simulink model "BLDC_Lun"  (R2021b)
settings: Solver=FixedStepAuto  StartTime=0.0  StopTime=10  FixedStep=1e-4  RelTol=1e-4
model workspace (MAT data in the model file):
  f = Simulink.Signal
  f.DataType = 'single'
  f.Dimensions = 1
  f.DimensionsMode = 'auto'
  f.Complexity = 'real'
  f.SampleTime = -1
  f.SamplingMode = 'auto'
  f.InitialValue = '0.1827'
undefined symbols (not defined in the file): curr_d_ki, curr_d_kp, curr_q_ki, curr_q_kp, DiscIntNeverNeededParam, flux, G1, G2, L, Pn, Rs, sigbuilder_block, spd_ki, spd_kp, Tpwm, Ts, Udc
libraries: slpidlib x4, simulink x2, mcbplantlib x1, autolibpmsmexterior x1
settings Model: DataDictionary=BLDC_Lun.sldd  PacingRate=0.630000  Creator=张豪  LastModifiedBy=张豪
settings OptimizationCC: DefaultParameterBehavior=Inlined  UseDivisionForNetSlopeComputation=on  GainParamInheritBuiltInType=on  UseFloatMulNetSlope=on  InlineInvariantSignals=on  PassReuseOutputArgsAs=Individual arguments  ZeroExternalMemoryAtStartup=off  ZeroInternalMemoryAtStartup=off  NoFixptDivByZeroProtection=on  EfficientFloat2IntCast=on  LifeSpan=1  OptimizeBlockOrder=speed  DifferentSizesBufferReuse=on  EfficientTunableParamExpr=on
settings DebuggingCC: ParameterTunabilityLossMsg=error
settings HardwareCC: ProdBitPerPointer=32  ProdBitPerSizeT=32  ProdBitPerPtrDiffT=32  ProdLargestAtomicInteger=Long  ProdLargestAtomicFloat=Double  ProdWordSize=32  ProdLongLongMode=on  ProdHWDeviceType=ARM Compatible->ARM Cortex-M
settings SFSimCC: MATLABDynamicMemAlloc=off
settings RTWCC: Description=Embedded Coder  SystemTargetFile=ert.tlc  GenCodeOnly=on  TemplateMakefile=ert_default_tmf  GenerateReport=on  LaunchReport=on  GenerateCodeReplacementReport=on
settings CodeAppCC: ForceParamTrailComments=on  IgnoreCustomStorageClasses=off  OperatorAnnotations=on  SimulinkDataObjDesc=on  SFDataObjDesc=on  CustomSymbolStrGlobalVar=rt$N$M  CustomSymbolStrType=$N$M  CustomSymbolStrFcn=$N$M$F  CustomSymbolStrMacro=$N$M  InsertBlockDesc=on
settings ERTTargetCC: TargetLangStandard=C99 (ISO)  CodeReplacementLibrary=ARM Cortex-M  GenerateSampleERTMain=on  IncludeMdlTerminateFcn=off  CombineSignalStateStructs=on  SupportComplex=off  SupportNonInlinedSFcns=on  InlinedParameterPlacement=NonHierarchical  ERTCustomFileTemplate=example_file_process.tlc  ERTFilePackagingFormat=CompactWithDataFile

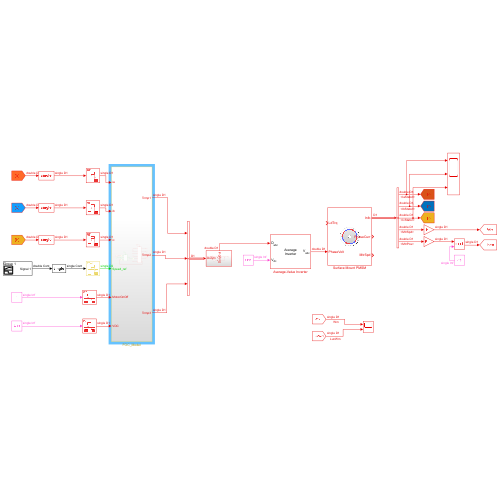
[thumbnail: Simulink's stored preview of the top-level diagram]
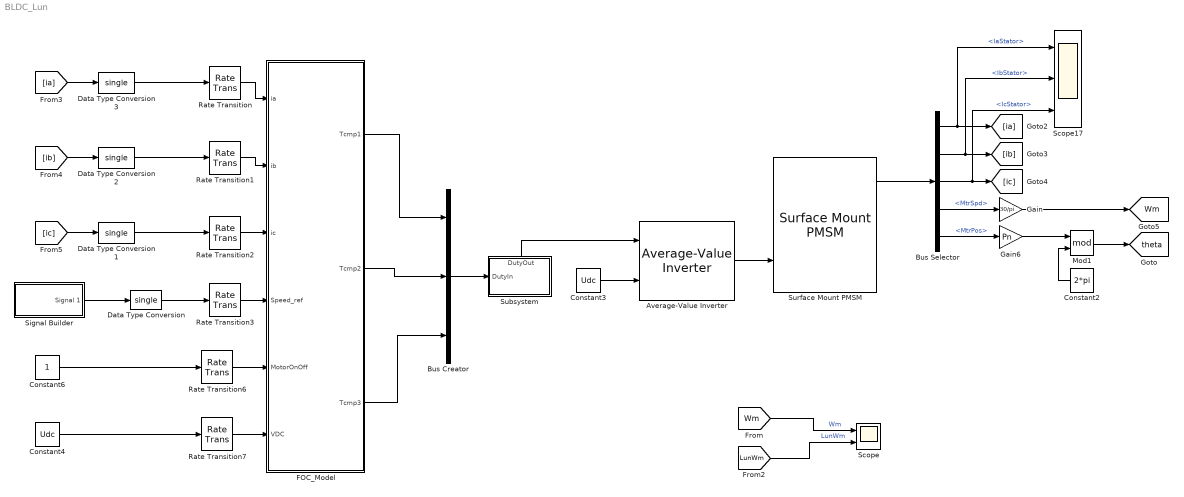
== system BLDC_Lun ==
  Average-Value Inverter : mcbplantlib/Average-Value Inverter
  Bus Creator : BusCreator  Inputs=3
  Bus Selector : BusSelector  OutputSignals=IaStator,IbStator,IcStator,MtrSpd,MtrPos
  Constant2 : Constant  Value=2*pi  OutDataTypeStr=single
  Constant3 : Constant  Value=Udc
  Constant4 : Constant  Value=Udc  OutDataTypeStr=single
  Constant6 : Constant  OutDataTypeStr=single
  Data Type Conversion{,1..3} (4 alike) : DataTypeConversion  OutDataTypeStr=single
  FOC_Model : Subsystem  SystemSampleTime=5e-5
  Gain : Gain  Gain=30/pi  OutDataTypeStr=single
  Gain6 : Gain  Gain=Pn  OutDataTypeStr=single
  Mod1 : Math  Operator=mod  OutputSignalType=real  SaturateOnIntegerOverflow=on
  Rate Transition{,1..3,6..7} (6 alike) : RateTransition
  Scope : Scope  NumInputPorts=2
  Scope17 : Scope  NumInputPorts=3
  Signal Builder : Subsystem  Tag=STV Subsys  LoadFcn=sigbuilder_block('load');  StartFcn=sigbuilder_block('start');  StopFcn=sigbuilder_block('stop');  ClipboardFcn=sigbuilder_block('clipboard');  mask(Sigbuilder block){tuvar=[0:10]}
      mask help: Simulink:masks:SigbuilderBlock_MD
      mask init:
      | if ~strcmp(get_param(bdroot(gcbh),'SimulationStatus'),'stopped') tuvar = sigbuilder_block('maskInit'); end
      settings: CopyFcn=sigbuilder_block('copy');  DeleteFcn=sigbuilder_block('delete');  ModelCloseFcn=sigbuilder_block('modelClose');  PreSaveFcn=sigbuilder_block('preSave');  PauseFcn=sigbuilder_block('pause');  ContinueFcn=sigbuilder_block('continue');  NameChangeFcn=sigbuilder_block('namechange');  OpenFcn=sigbuilder_block('open',[437.6 199.2 550.4 400 ]);  CloseFcn=sigbuilder_block('close');
      mask Display: plot(0, 0, 100, 100,[2, 2, 32, 32, 2], [68, 8, 8, 68, 68],[32, 2], [38, 38], [32, 19, 2],[53, 60, 44], [32, 17, 17, 2],[16, 16, 31, 31]);txt = getActiveGroup(gcbh);text(2, 100, txt,'verticalAlignment', 'top');
  Subsystem : Subsystem
      settings: PortSchema="{\"entries\":[{\"content\":{\"sides\":[{\"content\":{\"connectorIds\":[\"In1\"]},\"type\":\"ConnectorPlacement.EquallySpacedRectSide\",\"uuid\":\"8ccc51de-fa2a-4900-80a3-4cdf9aa76f01\"},{\"content\":{\"connectorIds\":[],\"side\":\"RIGHT\"},\"type\":\"ConnectorPlacement.EquallySpacedRectSide\",\"uuid\":\"32c06e0d-3f1d-4948-af96-e310e54308a0\"},{\"content\":{\"connectorIds\":[\"Out1\"],\"side\":\"TOP\"},\"type\":\"ConnectorPlacement.EquallySpacedRectSide\",\"uuid\":\"a9066067-2c54-42a8-b4d7-fb86ac71b860\"}]},\"type\":\"ConnectorPlacement.EquallySpacedConnector\",\"uuid\":\"e4576975-acad-4e16-822f-2c2e7f23d7a7\"}],\"packageUris\":[\"http://schema.mathworks.com/mf0/Connector/R2020b\"],\"version\":\"1.0\"}"
  Surface Mount PMSM : autolibpmsmexterior/Surface Mount PMSM  port_config=Torque  sim_type=Discrete  Ts=1e-4  P=Pn  Rs=Rs  Ldq_=L  KConstText=Permanent flux linkage constant (lambda_pm):  lambda_pm=flux  Ke=0.0059268  Kt=0.061  mechanical=[75e-6, 8e-5, 0]  idq0=[0 0]  theta_init=4/5  omega_init=0  KConst=flux  lambda_pm_calc=flux  RefBlkName='autolibpmsmexterior/Surface Mount PMSM'  aMode=5  Ldq="[0.0017      0.0017]"
      settings: SourceProductBaseCode=PW,DR,MT,UV,VE
  tag scope: Wm=global, theta=global
  wires:
  Gain/1 -> [Wm]
  [ia] -> Data Type Conversion3/1
  [ib] -> Data Type Conversion2/1
  [ic] -> Data Type Conversion1/1
  Subsystem/1(DutyOut) -> Average-Value Inverter/1
  Average-Value Inverter/1 -> Surface Mount PMSM/2
  Constant3/1 -> Average-Value Inverter/2
  Surface Mount PMSM/1 -> Bus Selector/1
  Bus Selector/1 -> Scope17/1, [ia]  "<IaStator>"
  Bus Selector/2 -> Scope17/2, [ib]  "<IbStator>"
  Bus Selector/3 -> Scope17/3, [ic]  "<IcStator>"
  Bus Selector/4 -> Gain/1  "<MtrSpd>"
  Bus Selector/5 -> Gain6/1  "<MtrPos>"
  Bus Creator/1 -> Subsystem/1(DutyIn)
  FOC_Model/1(Tcmp1) -> Bus Creator/1
  FOC_Model/2(Tcmp2) -> Bus Creator/2
  FOC_Model/3(Tcmp3) -> Bus Creator/3
  Data Type Conversion3/1 -> Rate Transition/1
  Data Type Conversion2/1 -> Rate Transition1/1
  Data Type Conversion1/1 -> Rate Transition2/1
  Signal Builder/1(Signal 1) -> Data Type Conversion/1
  Gain6/1 -> Mod1/1
  Constant2/1 -> Mod1/2
  Rate Transition/1 -> FOC_Model/1(ia)
  Rate Transition1/1 -> FOC_Model/2(ib)
  Rate Transition2/1 -> FOC_Model/3(ic)
  Rate Transition3/1 -> FOC_Model/4(Speed_ref)
  Data Type Conversion/1 -> Rate Transition3/1
  Constant4/1 -> Rate Transition7/1
  Rate Transition6/1 -> FOC_Model/5(MotorOnOff)
  Rate Transition7/1 -> FOC_Model/6(VDC)
  Constant6/1 -> Rate Transition6/1
  Mod1/1 -> [theta]
  [Wm] -> Scope/1  "Wm"
  [LunWm] -> Scope/2  "LunWm"

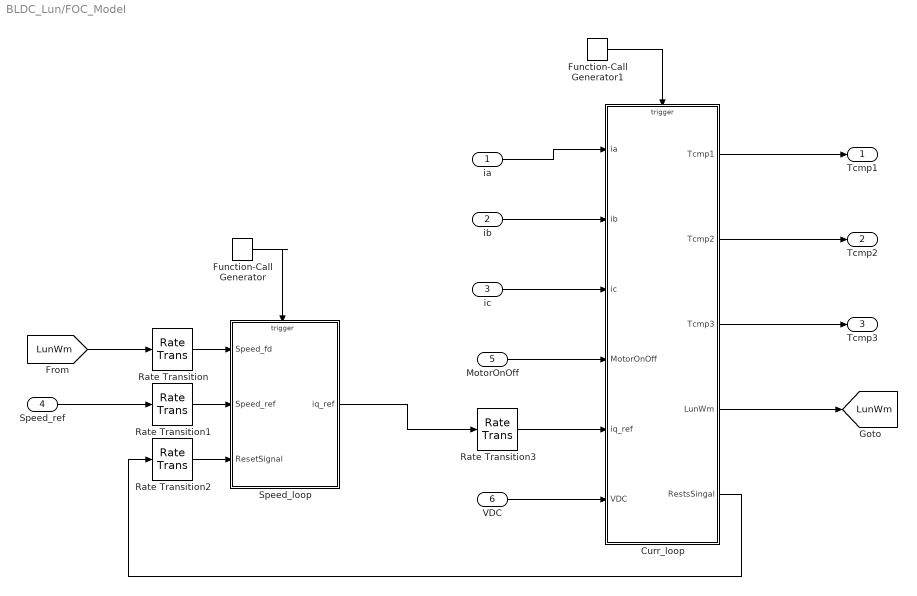
== system BLDC_Lun/FOC_Model ==
  ia : Inport
  ib : Inport  Port=2
  ic : Inport  Port=3
  Speed_ref : Inport  Port=4
  MotorOnOff : Inport  Port=5
  VDC : Inport  Port=6
  Curr_loop : Subsystem  TreatAsAtomicUnit=on
  Function-Call Generator : simulink/Ports & Subsystems/Function-Call Generator  sample_time=1e-3  numberOfIterations=1  DisallowWideOutput=off
  Function-Call Generator1 : simulink/Ports & Subsystems/Function-Call Generator  sample_time=1e-4  numberOfIterations=1  DisallowWideOutput=off
  Rate Transition{,1..3} (4 alike) : RateTransition
  Speed_loop : Subsystem
  Tcmp1 : Outport
  Tcmp2 : Outport  Port=2
  Tcmp3 : Outport  Port=3
  tag scope: LunWm=global
  wires:
  ia/1 -> Curr_loop/1(ia)
  Curr_loop/3(Tcmp3) -> Tcmp3/1
  Curr_loop/1(Tcmp1) -> Tcmp1/1
  ib/1 -> Curr_loop/2(ib)
  Curr_loop/2(Tcmp2) -> Tcmp2/1
  ic/1 -> Curr_loop/3(ic)
  Speed_ref/1 -> Rate Transition1/1
  MotorOnOff/1 -> Curr_loop/4(MotorOnOff)
  VDC/1 -> Curr_loop/6(VDC)
  Curr_loop/4(LunWm) -> [LunWm]
  Rate Transition/1 -> Speed_loop/1(Speed_fd)
  Rate Transition1/1 -> Speed_loop/2(Speed_ref)
  Rate Transition2/1 -> Speed_loop/3(ResetSignal)
  Curr_loop/5(RestsSingal) -> Rate Transition2/1
  [LunWm] -> Rate Transition/1
  Function-Call Generator/1 -> Speed_loop/Trigger
  Rate Transition3/1 -> Curr_loop/5(iq_ref)
  Function-Call Generator1/1 -> Curr_loop/Trigger
  Speed_loop/1(iq_ref) -> Rate Transition3/1

== system BLDC_Lun/Signal Builder ==
  Demux : Demux  Tag=STV Demux  Outputs=1
      settings: DisplayOption=none
  FromWs : FromWorkspace  Tag=STV FromWs  VariableName=tuvar
      SigBuilderData=|
      | common.afterFinalStr = 'Extrapolate'
      | common.sampleTime = 0
      | dataSet.timeRange = [0 10]
      | dataSet.name = 'Group 1'
      | sbobj.Groups.Name = 'Group 1'
      | sbobj.Groups.Signals.Name = 'Signal 1'
      | sbobj.Groups.Signals.XData = [0 4 4 7 7 10]
      | sbobj.Groups.Signals.YData = [680 680 1020 1020 1200 1200]
  Signal 1 : Outport  Tag=STV Outport
  wires:
  Demux/1 -> Signal 1/1
  FromWs/1 -> Demux/1

== system BLDC_Lun/Subsystem ==
  DutyIn : Inport
  Constant : Constant  Value=0.5  SampleTime=-1
  Gain : Gain  Gain=1/8000  ParamDataTypeStr=single
  Gain1 : Gain  Gain=-1
  Sum : Sum  Inputs=|+-
  Sum1 : Sum  Inputs=|++
  DutyOut : Outport
  wires:
  Sum/1 -> Gain1/1
  Constant/1 -> Sum1/2, Sum/2
  DutyIn/1 -> Gain/1
  Gain1/1 -> Sum1/1
  Sum1/1 -> DutyOut/1
  Gain/1 -> Sum/1

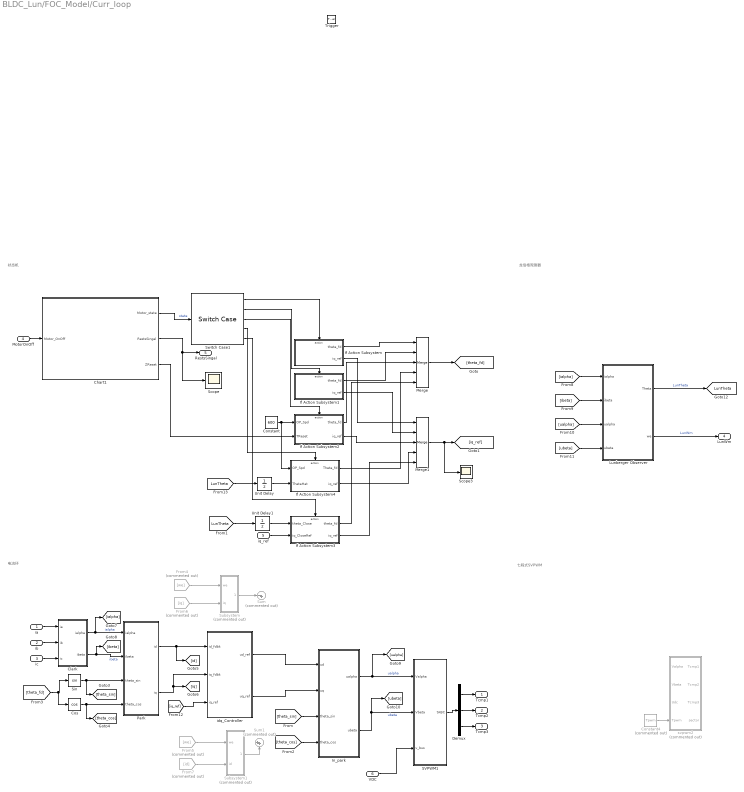
== system BLDC_Lun/FOC_Model/Curr_loop ==
  note: 七段式SVPWM
  note: 电流环
  note: 龙伯格观测器
  note: 状态机
  ia : Inport  OutDataTypeStr=single
  ib : Inport  Port=2  OutDataTypeStr=single
  ic : Inport  Port=3  OutDataTypeStr=single
  MotorOnOff : Inport  Port=4
  iq_ref : Inport  Port=5  OutDataTypeStr=single
  VDC : Inport  Port=6
  Trigger : TriggerPort  TriggerType=function-call  VariantControl=(inherit)  PortDimensions=1
  Chart1 : Stateflow chart  TreatAsAtomicUnit=on
  Clark : Subsystem  TreatAsAtomicUnit=on
  Constant : Constant  Value=600  OutDataTypeStr=int32
  Constant4 : Constant  Commented=on  Value=Tpwm  OutDataTypeStr=single
  Cos : Trigonometry  Operator=cos
  Demux : Demux  Outputs=3
  From4 : From  Commented=on  GotoTag=we
  From5 : From  Commented=on  GotoTag=we
  From6 : From  Commented=on  GotoTag=iq
  From7 : From  Commented=on  GotoTag=id
  If Action Subsystem : Subsystem  TreatAsAtomicUnit=on
  If Action Subsystem1 : Subsystem  TreatAsAtomicUnit=on
  If Action Subsystem2 : Subsystem  TreatAsAtomicUnit=on
  If Action Subsystem3 : Subsystem  TreatAsAtomicUnit=on
  If Action Subsystem4 : Subsystem  TreatAsAtomicUnit=on
  In_park : Subsystem  TreatAsAtomicUnit=on
  Lunberger Observer : Subsystem  TreatAsAtomicUnit=on
  Merge : Merge  Inputs=5
  Merge1 : Merge  Inputs=5
  Park : Subsystem  TreatAsAtomicUnit=on
  SVPWM1 : Subsystem  TreatAsAtomicUnit=on
  Scope : Scope
  Scope3 : Scope
  Sin : Trigonometry
  Subsystem : Subsystem  Commented=on
  Subsystem1 : Subsystem  Commented=on
  Sum : Sum  Commented=on  Inputs=|-+
  Sum1 : Sum  Commented=on  Inputs=|++
  Switch Case1 : SwitchCase  CaseConditions={1,2,3,4,5}  ShowDefaultCase=off
  Unit Delay : UnitDelay  SampleTime=-1  HasFrameUpgradeWarning=on
  Unit Delay1 : UnitDelay  SampleTime=-1  HasFrameUpgradeWarning=on
  idq_Controller : Subsystem
  svpwm2 : MATLAB Function  Commented=on  TreatAsAtomicUnit=on
  Tcmp1 : Outport
  Tcmp2 : Outport  Port=2
  Tcmp3 : Outport  Port=3
  LunWm : Outport  Port=4
  RestsSingal : Outport  Port=5
  tag scope: LunTheta=global
  wires:
  [iq_ref] -> idq_Controller/3(iq_ref)
  Clark/2(ibeta) -> [ibeta], Park/2(ibeta)  "ibeta"
  Park/1(id) -> [id], idq_Controller/1(id_fdbk)
  ib/1 -> Clark/2(ib)
  ia/1 -> Clark/1(ia)
  Clark/1(ialpha) -> [ialpha], Park/1(ialpha)  "ialpha"
  VDC/1 -> SVPWM1/3(v_bus)
  Park/2(iq) -> [iq], idq_Controller/2(iq_fdbk)
  Constant4/1 -> svpwm2/4(Tpwm)
  ic/1 -> Clark/3(ic)
  SVPWM1/1(tABC) -> Demux/1
  Demux/1 -> Tcmp1/1
  Demux/2 -> Tcmp2/1
  Demux/3 -> Tcmp3/1
  In_park/1(ualpha) -> [ualpha], SVPWM1/1(Valpha)  "ualpha"
  In_park/2(ubeta) -> [ubeta], SVPWM1/2(Vbeta)  "ubeta"
  MotorOnOff/1 -> Chart1/1(Motor_OnOff)
  Chart1/1(Motor_state) -> Switch Case1/1  "state"
  Switch Case1/1 -> If Action Subsystem/Action
  Switch Case1/2 -> If Action Subsystem1/Action
  Switch Case1/3 -> If Action Subsystem2/Action
  iq_ref/1 -> If Action Subsystem3/2(iq_CloseRef)
  Constant/1 -> If Action Subsystem4/1(OP_Spd), If Action Subsystem2/1(OP_Spd)
  Chart1/2(RestsSingal) -> Scope/1, RestsSingal/1
  If Action Subsystem/1(theta_fd) -> Merge/1
  If Action Subsystem1/1(theta_fd) -> Merge/2
  If Action Subsystem2/1(theta_fd) -> Merge/3
  If Action Subsystem/2(iq_ref) -> Merge1/1
  If Action Subsystem1/2(iq_ref) -> Merge1/2
  If Action Subsystem2/2(iq_ref) -> Merge1/3
  Merge/1 -> [theta_fd]
  Merge1/1 -> Scope3/1, [iq_ref]
  [LunTheta] -> Unit Delay1/1
  Subsystem/1(Out1) -> Sum/1
  Cos/1 -> [theta_cos], Park/4(theta_cos)
  Sin/1 -> Park/3(theta_sin), [theta_sin]
  Subsystem1/1(Out1) -> Sum1/2
  [theta_sin] -> In_park/3(theta_sin)
  [theta_cos] -> In_park/4(theta_cos)
  From4/1 -> Subsystem/1(we)
  From5/1 -> Subsystem1/1(we)
  From6/1 -> Subsystem/2(iq)
  From7/1 -> Subsystem1/2(id)
  [ialpha] -> Lunberger Observer/1(ialpha)
  [ibeta] -> Lunberger Observer/2(ibeta)
  [ualpha] -> Lunberger Observer/3(ualpha)
  [ubeta] -> Lunberger Observer/4(ubeta)
  Chart1/3(ZReset) -> If Action Subsystem2/2(TReset)
  [theta_fd] -> Cos/1, Sin/1
  idq_Controller/2(uq_ref) -> In_park/2(uq)
  idq_Controller/1(ud_ref) -> In_park/1(ud)
  Switch Case1/4 -> If Action Subsystem4/Action
  Switch Case1/5 -> If Action Subsystem3/Action
  If Action Subsystem3/1(theta_fd) -> Merge/5
  If Action Subsystem3/2(iq_ref) -> Merge1/5
  If Action Subsystem4/1(Theta_fd) -> Merge/4
  If Action Subsystem4/2(iq_ref) -> Merge1/4
  Lunberger Observer/1(Theta) -> [LunTheta]  "LunTheta"
  Lunberger Observer/2(we) -> LunWm/1  "LunWm"
  [LunTheta] -> Unit Delay/1
  Unit Delay/1 -> If Action Subsystem4/2(ThetaHat)
  Unit Delay1/1 -> If Action Subsystem3/1(theta_Close)

== system BLDC_Lun/FOC_Model/Speed_loop ==
  Speed_fd : Inport  OutDataTypeStr=single  PortDimensions=1
  Speed_ref : Inport  Port=2  OutDataTypeStr=single  PortDimensions=1
  ResetSignal : Inport  Port=3
  Trigger : TriggerPort  TriggerType=function-call  VariantControl=(inherit)  PortDimensions=1
  PID Controller3 : slpidlib/PID Controller  Controller=PI  Form=Parallel  TimeDomain=Discrete-time  UseExternalTs=off  SampleTime=-1  IntegratorMethod=Forward Euler  FilterMethod=Forward Euler  ControllerParametersSource=internal  P=spd_kp  I=spd_ki  D=0  UseFilter=on  N=100  TunerSelectOption=Transfer Function Based (PID Tuner App)  InitialConditionSource=internal  InitialConditionForIntegrator=0  InitialConditionForFilter=0  DifferentiatorICPrevScaledInput=0  ExternalReset=rising  TrackingMode=off  Kt=1  LimitOutput=on  SatLimitsSource=internal  UpperSaturationLimit=3  LowerSaturationLimit=-3  LinearizeAsGain=on  AntiWindupMode=clamping  Kb=0.013  PGainOutDataTypeStr=single  PProdOutDataTypeStr=single  POutMin=[]  POutMax=[]  IGainOutDataTypeStr=single  IProdOutDataTypeStr=single  IOutMin=[]  IOutMax=[]  DOutMin=[]  DOutMax=[]  NOutMin=[]  NOutMax=[]  SumOutDataTypeStr=single  SumOutMin=[]  SumOutMax=[]  SaturationOutDataTypeStr=single  SaturationOutMin=[]  SaturationOutMax=[]  PParamMin=[]  PParamMax=[]  IParamMin=[]  IParamMax=[]  DParamMin=[]  DParamMax=[]  NParamMin=[]  NParamMax=[]  KbParamMin=[]  KbParamMax=[]  KtParamMin=[]  KtParamMax=[]  KbOutMin=[]  KbOutMax=[]  KtOutMin=[]  KtOutMax=[]  IntegratorOutMin=[]  IntegratorOutMax=[]  FilterOutMin=[]  FilterOutMax=[]  SumI1OutMin=[]  SumI1OutMax=[]  SumI2OutMin=[]  SumI2OutMax=[]  SumI3OutMin=[]  SumI3OutMax=[]  SumI4OutMin=[]  SumI4OutMax=[]  SumDOutMin=[]  SumDOutMax=[]  DifferentiatorOutMin=[]  DifferentiatorOutMax=[]  FilterDiffOutCoefMin=[]  FilterDiffOutCoefMax=[]  ReciprocalOutMin=[]  ReciprocalOutMax=[]  SumDenOutMin=[]  SumDenOutMax=[]  SumNumOutMin=[]  SumNumOutMax=[]  DivideOutMin=[]  DivideOutMax=[]  UdiffTsProdOutMin=[]  UdiffTsProdOutMax=[]  NTsProdOutMin=[]  NTsProdOutMax=[]  UintegralTsProdOutMin=[]  UintegralTsProdOutMax=[]  UngainTsProdOutMin=[]  UngainTsProdOutMax=[]  IntegratorContinuousStateAttributes=''  IntegratorStateMustResolveToSignalObject=off  IntegratorRTWStateStorageClass=Auto  FilterContinuousStateAttributes=''  FilterStateMustResolveToSignalObject=off  FilterRTWStateStorageClass=Auto  ParallelPVariant=InternalParameters  IdealPVariant=Disabled  IVariant=InternalParameters  DVariant=Disabled  IntegratorVariant=Discrete  SatVariant=Enabled  AWVariant=DiscClampingParallel  PCopyVariant=Disabled  TRVariant=Disabled  FdbkBlocksVariant=Forward  IdealPFdbkVariant=Disabled  SatFdbkVariant=Disabled  DerivativeFilterVariant=Disabled  NVariant=Disabled  NCopyVariant=Disabled_SignalSpec  FilterICVariant=Disabled  IntegratorICVariant=InternalICs  ExternalResetVariant=ExternalReset  TRSumVariant=Passthrough  SumFdbkVariant=Disabled  SumVariant=Sum_PI  TsampFilterVariant=InternalTs  TsampNgainVariant=Passthrough  TsampIntegralVariant=Passthrough  ExternalSaturationOutDataTypeStr=single
  Sum2 : Sum  Inputs=|+-  AccumDataTypeStr=single  OutDataTypeStr=single
  iq_ref : Outport
  wires:
  Sum2/1 -> PID Controller3/1
  Speed_ref/1 -> Sum2/1
  Speed_fd/1 -> Sum2/2
  PID Controller3/1 -> iq_ref/1
  ResetSignal/1 -> PID Controller3/2

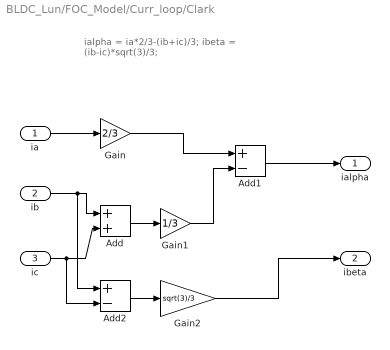
== system BLDC_Lun/FOC_Model/Curr_loop/Clark ==
  note: ialpha = ia*2/3-(ib+ic)/3;
      | ibeta = (ib-ic)*sqrt(3)/3;
  ia : Inport  OutDataTypeStr=single
  ib : Inport  Port=2  OutDataTypeStr=single
  ic : Inport  Port=3  OutDataTypeStr=single
  Add : Sum  AccumDataTypeStr=single  OutDataTypeStr=single
  Add1 : Sum  Inputs=+-  AccumDataTypeStr=single  OutDataTypeStr=single
  Add2 : Sum  Inputs=+-  AccumDataTypeStr=single  OutDataTypeStr=single
  Gain : Gain  Gain=2/3  ParamDataTypeStr=single
  Gain1 : Gain  Gain=1/3  ParamDataTypeStr=single
  Gain2 : Gain  Gain=sqrt(3)/3  ParamDataTypeStr=single
  ialpha : Outport  OutDataTypeStr=single
  ibeta : Outport  Port=2  OutDataTypeStr=single
  wires:
  ia/1 -> Gain/1
  ib/1 -> Add2/1, Add/1
  ic/1 -> Add2/2, Add/2
  Add/1 -> Gain1/1
  Gain/1 -> Add1/1
  Gain1/1 -> Add1/2
  Add1/1 -> ialpha/1
  Add2/1 -> Gain2/1
  Gain2/1 -> ibeta/1

== system BLDC_Lun/FOC_Model/Curr_loop/If Action Subsystem ==
  Action Port : ActionPort  ActionPortLabel=case [ 1 ]:
  Constant : Constant  Value=0  OutDataTypeStr=single
  Constant1 : Constant  Value=0  OutDataTypeStr=single
  theta_fd : Outport
  iq_ref : Outport  Port=2
  wires:
  Constant/1 -> theta_fd/1
  Constant1/1 -> iq_ref/1

== system BLDC_Lun/FOC_Model/Curr_loop/If Action Subsystem1 ==
  Action Port : ActionPort  ActionPortLabel=case [ 2 ]:
  Constant : Constant  Value=0  OutDataTypeStr=single
  Constant1 : Constant  OutDataTypeStr=single
  theta_fd : Outport
  iq_ref : Outport  Port=2
  wires:
  Constant1/1 -> iq_ref/1
  Constant/1 -> theta_fd/1

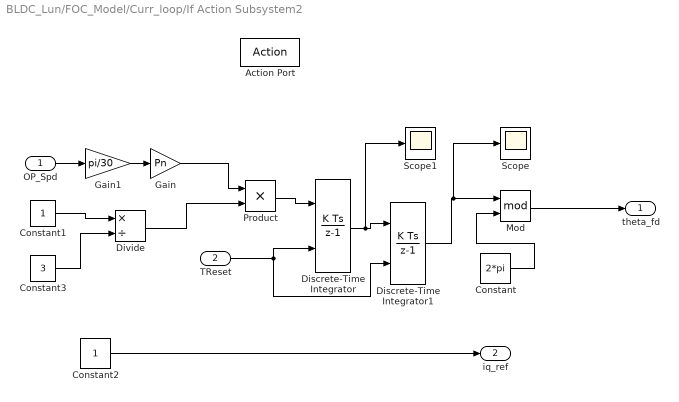
== system BLDC_Lun/FOC_Model/Curr_loop/If Action Subsystem2 ==
  OP_Spd : Inport  OutDataTypeStr=int32  PortDimensions=1
  TReset : Inport  Port=2
  Action Port : ActionPort  ActionPortLabel=case [ 3 ]:
  Constant : Constant  Value=2*pi  OutDataTypeStr=single
  Constant1 : Constant  OutDataTypeStr=single
  Constant2 : Constant  OutDataTypeStr=single
  Constant3 : Constant  Value=3  OutDataTypeStr=single
  Discrete-Time Integrator : DiscreteIntegrator  ExternalReset=rising  SampleTime=-1  ICPrevOutput=DiscIntNeverNeededParam  ICPrevScaledInput=DiscIntNeverNeededParam
  Discrete-Time Integrator1 : DiscreteIntegrator  ExternalReset=rising  SampleTime=-1  ICPrevOutput=DiscIntNeverNeededParam  ICPrevScaledInput=DiscIntNeverNeededParam
  Divide : Product  Inputs=*/  OutDataTypeStr=single
  Gain : Gain  Gain=Pn
  Gain1 : Gain  Gain=pi/30  OutDataTypeStr=single
  Mod : Math  Operator=mod  SaturateOnIntegerOverflow=on
  Product : Product  OutDataTypeStr=single
  Scope : Scope
  Scope1 : Scope
  theta_fd : Outport
  iq_ref : Outport  Port=2
  wires:
  Gain1/1 -> Gain/1
  Constant1/1 -> Divide/1
  Gain/1 -> Product/1
  Constant/1 -> Mod/2
  Discrete-Time Integrator1/1 -> Scope/1, Mod/1
  Mod/1 -> theta_fd/1
  Constant3/1 -> Divide/2
  Constant2/1 -> iq_ref/1
  Divide/1 -> Product/2
  Product/1 -> Discrete-Time Integrator/1
  OP_Spd/1 -> Gain1/1
  TReset/1 -> Discrete-Time Integrator/2, Discrete-Time Integrator1/2
  Discrete-Time Integrator/1 -> Scope1/1, Discrete-Time Integrator1/1

== system BLDC_Lun/FOC_Model/Curr_loop/If Action Subsystem3 ==
  theta_Close : Inport
  iq_CloseRef : Inport  Port=2
  Action Port : ActionPort  ActionPortLabel=case [ 5 ]:
  theta_fd : Outport
  iq_ref : Outport  Port=2
  wires:
  iq_CloseRef/1 -> iq_ref/1
  theta_Close/1 -> theta_fd/1

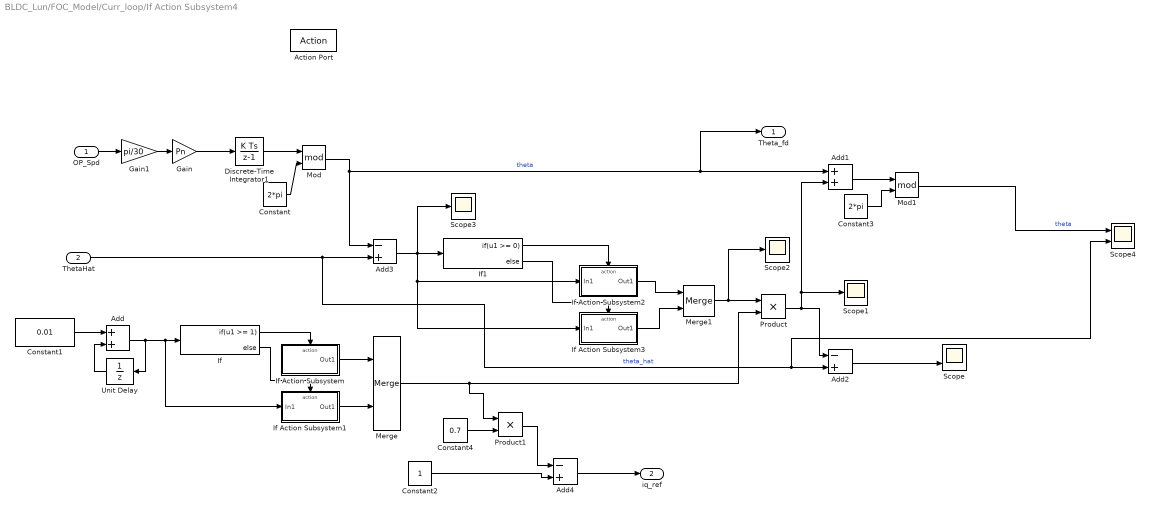
== system BLDC_Lun/FOC_Model/Curr_loop/If Action Subsystem4 ==
  OP_Spd : Inport  OutDataTypeStr=int32  PortDimensions=1
  ThetaHat : Inport  Port=2
  Action Port : ActionPort  ActionPortLabel=case [ 4 ]:
  Add : Sum
  Add1 : Sum
  Add2 : Sum  Inputs=-+
  Add3 : Sum  Inputs=-+
  Add4 : Sum  Inputs=-+
  Constant : Constant  Value=2*pi  OutDataTypeStr=single
  Constant1 : Constant  Value=0.01  OutDataTypeStr=single
  Constant2 : Constant  OutDataTypeStr=single
  Constant3 : Constant  Value=2*pi  OutDataTypeStr=single
  Constant4 : Constant  Value=0.7  OutDataTypeStr=single
  Discrete-Time Integrator1 : DiscreteIntegrator  SampleTime=-1  ICPrevOutput=DiscIntNeverNeededParam  ICPrevScaledInput=DiscIntNeverNeededParam
  Gain : Gain  Gain=Pn
  Gain1 : Gain  Gain=pi/30  OutDataTypeStr=single
  If : If  IfExpression=u1 >= 1
  If Action Subsystem : Subsystem  TreatAsAtomicUnit=on
  If Action Subsystem1 : Subsystem  TreatAsAtomicUnit=on
  If Action Subsystem2 : Subsystem  TreatAsAtomicUnit=on
  If Action Subsystem3 : Subsystem  TreatAsAtomicUnit=on
  If1 : If  IfExpression=u1 >= 0
  Merge : Merge
  Merge1 : Merge
  Mod : Math  Operator=mod  SaturateOnIntegerOverflow=on
  Mod1 : Math  Operator=mod  SaturateOnIntegerOverflow=on
  Product : Product
  Product1 : Product
  Scope : Scope  NumInputPorts=2
  Scope1 : Scope
  Scope2 : Scope
  Scope3 : Scope
  Scope4 : Scope  NumInputPorts=2
  Unit Delay : UnitDelay  SampleTime=-1  HasFrameUpgradeWarning=on
  Theta_fd : Outport
  iq_ref : Outport  Port=2
  wires:
  Gain/1 -> Discrete-Time Integrator1/1
  Constant/1 -> Mod/2
  Discrete-Time Integrator1/1 -> Mod/1
  Constant1/1 -> Add/1
  OP_Spd/1 -> Gain1/1
  If/1 -> If Action Subsystem/Action
  Gain1/1 -> Gain/1
  If Action Subsystem1/1(Out1) -> Merge/2
  Unit Delay/1 -> Add/2
  Add/1 -> Unit Delay/1, If/1, If Action Subsystem1/1(In1)
  If Action Subsystem/1(Out1) -> Merge/1
  If/2 -> If Action Subsystem1/Action
  ThetaHat/1 -> Scope4/2, Add2/2, Add3/2  "theta_hat"
  Mod/1 -> Theta_fd/1, Add1/1, Add3/1  "theta"
  Add3/1 -> Scope3/1, If Action Subsystem3/1(In1), If Action Subsystem2/1(In1), If1/1
  If1/1 -> If Action Subsystem2/Action
  If1/2 -> If Action Subsystem3/Action
  If Action Subsystem2/1(Out1) -> Merge1/1
  If Action Subsystem3/1(Out1) -> Merge1/2
  Merge1/1 -> Scope2/1, Product/1
  Merge/1 -> Product1/1, Product/2
  Product/1 -> Add1/2, Scope1/1, Add2/1
  Add2/1 -> Scope/2
  Constant3/1 -> Mod1/2
  Add1/1 -> Mod1/1
  Mod1/1 -> Scope4/1  "theta"
  Constant4/1 -> Product1/2
  Constant2/1 -> Add4/2
  Product1/1 -> Add4/1
  Add4/1 -> iq_ref/1

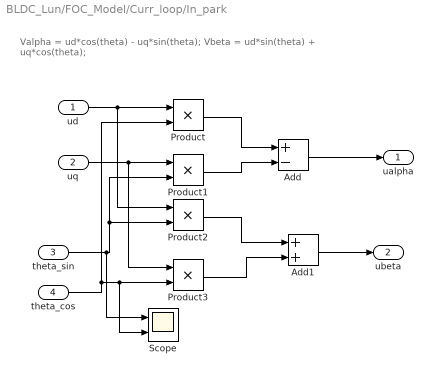
== system BLDC_Lun/FOC_Model/Curr_loop/In_park ==
  note: Valpha = ud*cos(theta) - uq*sin(theta);
      | Vbeta = ud*sin(theta) + uq*cos(theta);
  ud : Inport
  uq : Inport  Port=2
  theta_sin : Inport  Port=3
  theta_cos : Inport  Port=4
  Add : Sum  Inputs=+-
  Add1 : Sum
  Product{,1..3} (4 alike) : Product
  Scope : Scope  NumInputPorts=2
  ualpha : Outport
  ubeta : Outport  Port=2
  wires:
  Add/1 -> ualpha/1
  ud/1 -> Product2/1, Product/1
  theta_cos/1 -> Product/2, Scope/2, Product3/2
  Product/1 -> Add/1
  uq/1 -> Product3/1, Product1/1
  theta_sin/1 -> Scope/1, Product2/2, Product1/2
  Product1/1 -> Add/2
  Product2/1 -> Add1/1
  Product3/1 -> Add1/2
  Add1/1 -> ubeta/1

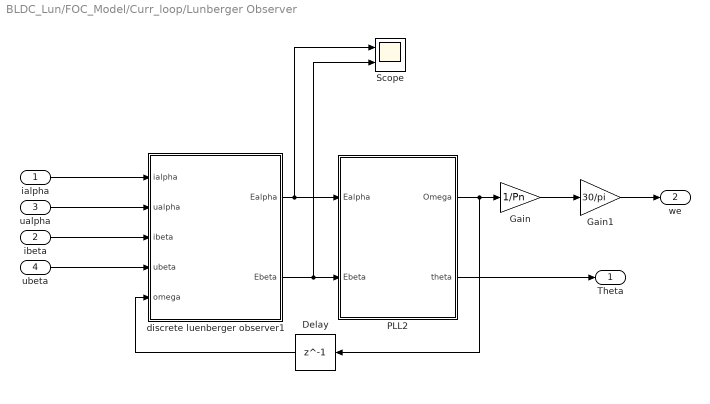
== system BLDC_Lun/FOC_Model/Curr_loop/Lunberger Observer ==
  ialpha : Inport  OutDataTypeStr=single
  ibeta : Inport  Port=2  OutDataTypeStr=single
  ualpha : Inport  Port=3  OutDataTypeStr=single
  ubeta : Inport  Port=4  OutDataTypeStr=single
  Delay : Delay  DelayLength=1  InputProcessing=Columns as channels (frame based)
  Gain : Gain  Gain=1/Pn
  Gain1 : Gain  Gain=30/pi
  PLL2 : Subsystem
  Scope : Scope  NumInputPorts=2
  discrete luenberger observer1 : Subsystem
  Theta : Outport
  we : Outport  Port=2
  wires:
  PLL2/2(theta) -> Theta/1
  ubeta/1 -> discrete luenberger observer1/4(ubeta)
  ibeta/1 -> discrete luenberger observer1/3(ibeta)
  ualpha/1 -> discrete luenberger observer1/2(ualpha)
  ialpha/1 -> discrete luenberger observer1/1(ialpha)
  Delay/1 -> discrete luenberger observer1/5(omega)
  discrete luenberger observer1/1(Ealpha) -> Scope/1, PLL2/1(Ealpha)
  discrete luenberger observer1/2(Ebeta) -> Scope/2, PLL2/2(Ebeta)
  PLL2/1(Omega) -> Gain/1, Delay/1
  Gain/1 -> Gain1/1
  Gain1/1 -> we/1

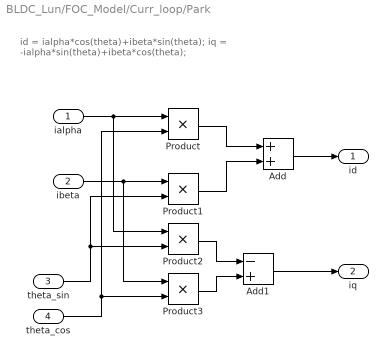
== system BLDC_Lun/FOC_Model/Curr_loop/Park ==
  note: id = ialpha*cos(theta)+ibeta*sin(theta);
      | iq = -ialpha*sin(theta)+ibeta*cos(theta);
  ialpha : Inport  OutDataTypeStr=single
  ibeta : Inport  Port=2  OutDataTypeStr=single
  theta_sin : Inport  Port=3  OutDataTypeStr=single
  theta_cos : Inport  Port=4  OutDataTypeStr=single
  Add : Sum  AccumDataTypeStr=single  OutDataTypeStr=single
  Add1 : Sum  Inputs=-+  AccumDataTypeStr=single  OutDataTypeStr=single
  Product{,1..3} (4 alike) : Product  OutDataTypeStr=single
  id : Outport  OutDataTypeStr=single
  iq : Outport  Port=2  OutDataTypeStr=single
  wires:
  ialpha/1 -> Product2/1, Product/1
  theta_cos/1 -> Product3/2, Product/2
  ibeta/1 -> Product3/1, Product1/1
  theta_sin/1 -> Product2/2, Product1/2
  Product/1 -> Add/1
  Product1/1 -> Add/2
  Add/1 -> id/1
  Product2/1 -> Add1/1
  Product3/1 -> Add1/2
  Add1/1 -> iq/1

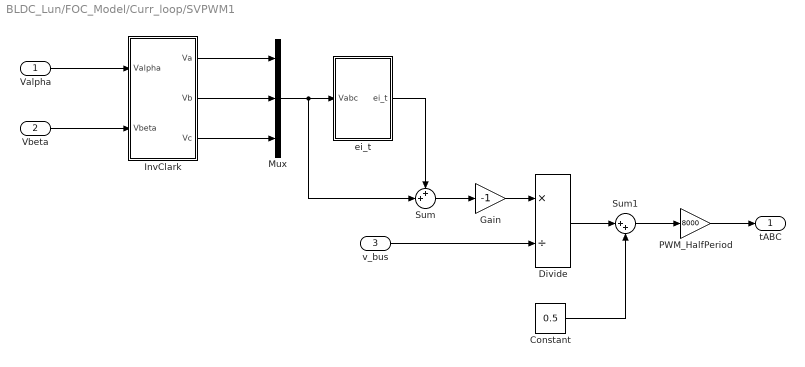
== system BLDC_Lun/FOC_Model/Curr_loop/SVPWM1 ==
  Valpha : Inport  OutDataTypeStr=single
  Vbeta : Inport  Port=2  OutDataTypeStr=single
  v_bus : Inport  Port=3  OutDataTypeStr=single
  Constant : Constant  Value=0.5  OutDataTypeStr=single
  Divide : Product  Inputs=*/  OutDataTypeStr=single
  Gain : Gain  Gain=-1  OutDataTypeStr=single
  InvClark : Subsystem
  Mux : Mux  Inputs=3
  PWM_HalfPeriod : Gain  Gain=8000  OutDataTypeStr=single
  Sum : Sum  Inputs=++|  OutDataTypeStr=single
  Sum1 : Sum  Inputs=|++  OutDataTypeStr=single
  ei_t : Subsystem
  tABC : Outport  OutDataTypeStr=single
  wires:
  Valpha/1 -> InvClark/1(Valpha)
  Vbeta/1 -> InvClark/2(Vbeta)
  ei_t/1(ei_t) -> Sum/1
  InvClark/1(Va) -> Mux/1
  InvClark/2(Vb) -> Mux/2
  InvClark/3(Vc) -> Mux/3
  Sum/1 -> Gain/1
  Mux/1 -> Sum/2, ei_t/1(Vabc)
  Divide/1 -> Sum1/1
  Constant/1 -> Sum1/2
  Sum1/1 -> PWM_HalfPeriod/1
  PWM_HalfPeriod/1 -> tABC/1
  v_bus/1 -> Divide/2
  Gain/1 -> Divide/1

== system BLDC_Lun/FOC_Model/Curr_loop/Subsystem ==
  we : Inport
  iq : Inport  Port=2
  Constant : Constant  Value=L  OutDataTypeStr=single
  Product : Product  Inputs=3
  Out1 : Outport
  wires:
  iq/1 -> Product/2
  we/1 -> Product/1
  Constant/1 -> Product/3
  Product/1 -> Out1/1

== system BLDC_Lun/FOC_Model/Curr_loop/Subsystem1 ==
  we : Inport
  id : Inport  Port=2
  Add : Sum
  Constant : Constant  Value=L  OutDataTypeStr=single
  Constant1 : Constant  Value=flux  OutDataTypeStr=single
  Product : Product
  Product1 : Product
  Out1 : Outport
  wires:
  id/1 -> Product/1
  Constant/1 -> Product/2
  Product/1 -> Add/2
  Constant1/1 -> Add/1
  Product1/1 -> Out1/1
  Add/1 -> Product1/2
  we/1 -> Product1/1

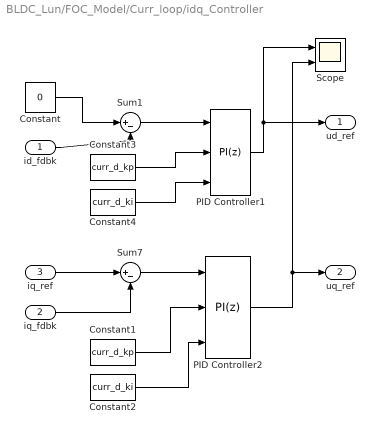
== system BLDC_Lun/FOC_Model/Curr_loop/idq_Controller ==
  id_fdbk : Inport  OutDataTypeStr=single
  iq_fdbk : Inport  Port=2  OutDataTypeStr=single
  iq_ref : Inport  Port=3  OutDataTypeStr=single
  Constant : Constant  Value=0  OutDataTypeStr=single
  Constant1 : Constant  Value=curr_d_kp  OutDataTypeStr=single
  Constant2 : Constant  Value=curr_d_ki  OutDataTypeStr=single
  Constant3 : Constant  Value=curr_d_kp  OutDataTypeStr=single
  Constant4 : Constant  Value=curr_d_ki  OutDataTypeStr=single
  PID Controller1 : slpidlib/PID Controller  Controller=PI  Form=Parallel  TimeDomain=Discrete-time  UseExternalTs=off  SampleTime=-1  IntegratorMethod=Forward Euler  FilterMethod=Forward Euler  ControllerParametersSource=external  P=curr_d_kp  I=curr_d_ki  D=0  UseFilter=on  N=100  TunerSelectOption=Transfer Function Based (PID Tuner App)  InitialConditionSource=internal  InitialConditionForIntegrator=0  InitialConditionForFilter=0  DifferentiatorICPrevScaledInput=0  ExternalReset=none  TrackingMode=off  Kt=1  LimitOutput=on  SatLimitsSource=internal  UpperSaturationLimit=24*0.9/sqrt(3)  LowerSaturationLimit=-24*0.9/sqrt(3)  LinearizeAsGain=on  AntiWindupMode=clamping  Kb=1  PGainOutDataTypeStr=single  PProdOutDataTypeStr=single  POutMin=[]  POutMax=[]  IGainOutDataTypeStr=int16  IProdOutDataTypeStr=int16  IOutMin=[]  IOutMax=[]  DOutMin=[]  DOutMax=[]  NOutMin=[]  NOutMax=[]  SumOutDataTypeStr=single  SumOutMin=[]  SumOutMax=[]  SaturationOutDataTypeStr=single  SaturationOutMin=[]  SaturationOutMax=[]  PParamMin=[]  PParamMax=[]  IParamMin=[]  IParamMax=[]  DParamMin=[]  DParamMax=[]  NParamMin=[]  NParamMax=[]  KbParamMin=[]  KbParamMax=[]  KtParamMin=[]  KtParamMax=[]  KbOutMin=[]  KbOutMax=[]  KtOutMin=[]  KtOutMax=[]  IntegratorOutMin=[]  IntegratorOutMax=[]  FilterOutMin=[]  FilterOutMax=[]  SumI1OutMin=[]  SumI1OutMax=[]  SumI2OutMin=[]  SumI2OutMax=[]  SumI3OutMin=[]  SumI3OutMax=[]  SumI4OutMin=[]  SumI4OutMax=[]  SumDOutMin=[]  SumDOutMax=[]  DifferentiatorOutMin=[]  DifferentiatorOutMax=[]  FilterDiffOutCoefMin=[]  FilterDiffOutCoefMax=[]  ReciprocalOutMin=[]  ReciprocalOutMax=[]  SumDenOutMin=[]  SumDenOutMax=[]  SumNumOutMin=[]  SumNumOutMax=[]  DivideOutMin=[]  DivideOutMax=[]  UdiffTsProdOutMin=[]  UdiffTsProdOutMax=[]  NTsProdOutMin=[]  NTsProdOutMax=[]  UintegralTsProdOutMin=[]  UintegralTsProdOutMax=[]  UngainTsProdOutMin=[]  UngainTsProdOutMax=[]  IntegratorContinuousStateAttributes=''  IntegratorStateMustResolveToSignalObject=off  IntegratorRTWStateStorageClass=Auto  FilterContinuousStateAttributes=''  FilterStateMustResolveToSignalObject=off  FilterRTWStateStorageClass=Auto  ParallelPVariant=ExternalParameters  IdealPVariant=Disabled  IVariant=ExternalParameters  DVariant=Disabled  IntegratorVariant=Discrete  SatVariant=Enabled  AWVariant=DiscClampingParallel  PCopyVariant=Disabled  TRVariant=Disabled  FdbkBlocksVariant=Forward  IdealPFdbkVariant=Disabled  SatFdbkVariant=Disabled  DerivativeFilterVariant=Disabled  NVariant=Disabled  NCopyVariant=Disabled_SignalSpec  FilterICVariant=Disabled  IntegratorICVariant=InternalICs  ExternalResetVariant=Disabled  TRSumVariant=Passthrough  SumFdbkVariant=Disabled  SumVariant=Sum_PI  TsampFilterVariant=InternalTs  TsampNgainVariant=Passthrough  TsampIntegralVariant=Passthrough  ExternalSaturationOutDataTypeStr=Inherit: Same as second input
  PID Controller2 : slpidlib/PID Controller  Controller=PI  Form=Parallel  TimeDomain=Discrete-time  UseExternalTs=off  SampleTime=-1  IntegratorMethod=Forward Euler  FilterMethod=Forward Euler  ControllerParametersSource=external  P=curr_q_kp  I=curr_q_ki  D=0  UseFilter=on  N=100  TunerSelectOption=Transfer Function Based (PID Tuner App)  InitialConditionSource=internal  InitialConditionForIntegrator=0  InitialConditionForFilter=0  DifferentiatorICPrevScaledInput=0  ExternalReset=none  TrackingMode=off  Kt=1  LimitOutput=on  SatLimitsSource=internal  UpperSaturationLimit=24*0.9/sqrt(3)  LowerSaturationLimit=-24*0.9/sqrt(3)  LinearizeAsGain=on  AntiWindupMode=clamping  Kb=1  PGainOutDataTypeStr=single  PProdOutDataTypeStr=single  POutMin=[]  POutMax=[]  IGainOutDataTypeStr=single  IProdOutDataTypeStr=single  IOutMin=[]  IOutMax=[]  DOutMin=[]  DOutMax=[]  NOutMin=[]  NOutMax=[]  SumOutDataTypeStr=single  SumOutMin=[]  SumOutMax=[]  SaturationOutDataTypeStr=single  SaturationOutMin=[]  SaturationOutMax=[]  PParamMin=[]  PParamMax=[]  IParamMin=[]  IParamMax=[]  DParamMin=[]  DParamMax=[]  NParamMin=[]  NParamMax=[]  KbParamMin=[]  KbParamMax=[]  KtParamMin=[]  KtParamMax=[]  KbOutMin=[]  KbOutMax=[]  KtOutMin=[]  KtOutMax=[]  IntegratorOutMin=[]  IntegratorOutMax=[]  FilterOutMin=[]  FilterOutMax=[]  SumI1OutMin=[]  SumI1OutMax=[]  SumI2OutMin=[]  SumI2OutMax=[]  SumI3OutMin=[]  SumI3OutMax=[]  SumI4OutMin=[]  SumI4OutMax=[]  SumDOutMin=[]  SumDOutMax=[]  DifferentiatorOutMin=[]  DifferentiatorOutMax=[]  FilterDiffOutCoefMin=[]  FilterDiffOutCoefMax=[]  ReciprocalOutMin=[]  ReciprocalOutMax=[]  SumDenOutMin=[]  SumDenOutMax=[]  SumNumOutMin=[]  SumNumOutMax=[]  DivideOutMin=[]  DivideOutMax=[]  UdiffTsProdOutMin=[]  UdiffTsProdOutMax=[]  NTsProdOutMin=[]  NTsProdOutMax=[]  UintegralTsProdOutMin=[]  UintegralTsProdOutMax=[]  UngainTsProdOutMin=[]  UngainTsProdOutMax=[]  IntegratorContinuousStateAttributes=''  IntegratorStateMustResolveToSignalObject=off  IntegratorRTWStateStorageClass=Auto  FilterContinuousStateAttributes=''  FilterStateMustResolveToSignalObject=off  FilterRTWStateStorageClass=Auto  ParallelPVariant=ExternalParameters  IdealPVariant=Disabled  IVariant=ExternalParameters  DVariant=Disabled  IntegratorVariant=Discrete  SatVariant=Enabled  AWVariant=DiscClampingParallel  PCopyVariant=Disabled  TRVariant=Disabled  FdbkBlocksVariant=Forward  IdealPFdbkVariant=Disabled  SatFdbkVariant=Disabled  DerivativeFilterVariant=Disabled  NVariant=Disabled  NCopyVariant=Disabled_SignalSpec  FilterICVariant=Disabled  IntegratorICVariant=InternalICs  ExternalResetVariant=Disabled  TRSumVariant=Passthrough  SumFdbkVariant=Disabled  SumVariant=Sum_PI  TsampFilterVariant=InternalTs  TsampNgainVariant=Passthrough  TsampIntegralVariant=Passthrough  ExternalSaturationOutDataTypeStr=Inherit: Same as second input
  Scope : Scope  NumInputPorts=2
  Sum1 : Sum  Inputs=|+-  AccumDataTypeStr=single  OutDataTypeStr=single
  Sum7 : Sum  Inputs=|+-  AccumDataTypeStr=single  OutDataTypeStr=single
  ud_ref : Outport  OutDataTypeStr=single
  uq_ref : Outport  Port=2  OutDataTypeStr=single
  wires:
  id_fdbk/1 -> Sum1/2
  Constant/1 -> Sum1/1
  iq_fdbk/1 -> Sum7/2
  Sum1/1 -> PID Controller1/1
  Sum7/1 -> PID Controller2/1
  PID Controller1/1 -> Scope/1, ud_ref/1
  PID Controller2/1 -> Scope/2, uq_ref/1
  iq_ref/1 -> Sum7/1
  Constant3/1 -> PID Controller1/2
  Constant4/1 -> PID Controller1/3
  Constant1/1 -> PID Controller2/2
  Constant2/1 -> PID Controller2/3

== system BLDC_Lun/FOC_Model/Curr_loop/If Action Subsystem4/If Action Subsystem ==
  Action Port : ActionPort  ActionPortLabel=if(u1 >= 1)
  Constant : Constant  OutDataTypeStr=single
  Out1 : Outport
  wires:
  Constant/1 -> Out1/1

== system BLDC_Lun/FOC_Model/Curr_loop/If Action Subsystem4/If Action Subsystem1 ==
  In1 : Inport
  Action Port : ActionPort  ActionPortLabel=else
  Out1 : Outport
  wires:
  In1/1 -> Out1/1

== system BLDC_Lun/FOC_Model/Curr_loop/If Action Subsystem4/If Action Subsystem2 ==
  In1 : Inport
  Action Port : ActionPort  ActionPortLabel=if(u1 >= 0)
  Out1 : Outport
  wires:
  In1/1 -> Out1/1

== system BLDC_Lun/FOC_Model/Curr_loop/If Action Subsystem4/If Action Subsystem3 ==
  In1 : Inport
  Action Port : ActionPort  ActionPortLabel=else
  Add : Sum
  Constant : Constant  Value=2*pi  OutDataTypeStr=single
  Out1 : Outport
  wires:
  In1/1 -> Add/1
  Constant/1 -> Add/2
  Add/1 -> Out1/1

== system BLDC_Lun/FOC_Model/Curr_loop/Lunberger Observer/PLL2 ==
  Ealpha : Inport
  Ebeta : Inport  Port=2
  Add8 : Sum  Inputs=--
  Cos : Trigonometry
  PID Controller : slpidlib/PID Controller  Controller=PI  Form=Parallel  TimeDomain=Discrete-time  UseExternalTs=off  SampleTime=-1  IntegratorMethod=Forward Euler  FilterMethod=Forward Euler  ControllerParametersSource=internal  P=2*0.707*150  I=50*50  D=0  UseFilter=on  N=100  TunerSelectOption=Transfer Function Based (PID Tuner App)  InitialConditionSource=internal  InitialConditionForIntegrator=0  InitialConditionForFilter=0  DifferentiatorICPrevScaledInput=0  ExternalReset=none  TrackingMode=off  Kt=1  LimitOutput=on  SatLimitsSource=internal  UpperSaturationLimit=2*pi*1000  LowerSaturationLimit=-2*pi*1000  LinearizeAsGain=on  AntiWindupMode=clamping  Kb=1  POutMin=[]  POutMax=[]  IOutMin=[]  IOutMax=[]  DOutMin=[]  DOutMax=[]  NOutMin=[]  NOutMax=[]  SumOutMin=[]  SumOutMax=[]  SaturationOutMin=[]  SaturationOutMax=[]  PParamMin=[]  PParamMax=[]  IParamMin=[]  IParamMax=[]  DParamMin=[]  DParamMax=[]  NParamMin=[]  NParamMax=[]  KbParamMin=[]  KbParamMax=[]  KtParamMin=[]  KtParamMax=[]  KbOutMin=[]  KbOutMax=[]  KtOutMin=[]  KtOutMax=[]  IntegratorOutMin=[]  IntegratorOutMax=[]  FilterOutMin=[]  FilterOutMax=[]  SumI1OutMin=[]  SumI1OutMax=[]  SumI2OutMin=[]  SumI2OutMax=[]  SumI3OutMin=[]  SumI3OutMax=[]  SumI4OutMin=[]  SumI4OutMax=[]  SumDOutMin=[]  SumDOutMax=[]  DifferentiatorOutMin=[]  DifferentiatorOutMax=[]  FilterDiffOutCoefMin=[]  FilterDiffOutCoefMax=[]  ReciprocalOutMin=[]  ReciprocalOutMax=[]  SumDenOutMin=[]  SumDenOutMax=[]  SumNumOutMin=[]  SumNumOutMax=[]  DivideOutMin=[]  DivideOutMax=[]  UdiffTsProdOutMin=[]  UdiffTsProdOutMax=[]  NTsProdOutMin=[]  NTsProdOutMax=[]  UintegralTsProdOutMin=[]  UintegralTsProdOutMax=[]  UngainTsProdOutMin=[]  UngainTsProdOutMax=[]  IntegratorContinuousStateAttributes=''  IntegratorStateMustResolveToSignalObject=off  IntegratorRTWStateStorageClass=Auto  FilterContinuousStateAttributes=''  FilterStateMustResolveToSignalObject=off  FilterRTWStateStorageClass=Auto  ParallelPVariant=InternalParameters  IdealPVariant=Disabled  IVariant=InternalParameters  DVariant=Disabled  IntegratorVariant=Discrete  SatVariant=Enabled  AWVariant=DiscClampingParallel  PCopyVariant=Disabled  TRVariant=Disabled  FdbkBlocksVariant=Forward  IdealPFdbkVariant=Disabled  SatFdbkVariant=Disabled  DerivativeFilterVariant=Disabled  NVariant=Disabled  NCopyVariant=Disabled_SignalSpec  FilterICVariant=Disabled  IntegratorICVariant=InternalICs  ExternalResetVariant=Disabled  TRSumVariant=Passthrough  SumFdbkVariant=Disabled  SumVariant=Sum_PI  TsampFilterVariant=InternalTs  TsampNgainVariant=Passthrough  TsampIntegralVariant=Passthrough  ExternalSaturationOutDataTypeStr=Inherit: Same as second input
  Product4 : Product
  Product5 : Product
  Sin : Trigonometry  Operator=cos
  SpeedToTheta : Subsystem
  Omega : Outport
  theta : Outport  Port=2
  wires:
  Product4/1 -> Add8/1
  Product5/1 -> Add8/2
  SpeedToTheta/1(Theta) -> theta/1, Cos/1, Sin/1  "theta"
  Ebeta/1 -> Product5/1
  Ealpha/1 -> Product4/1
  PID Controller/1 -> SpeedToTheta/1(we), Omega/1  "Omega"
  Sin/1 -> Product4/2
  Cos/1 -> Product5/2
  Add8/1 -> PID Controller/1

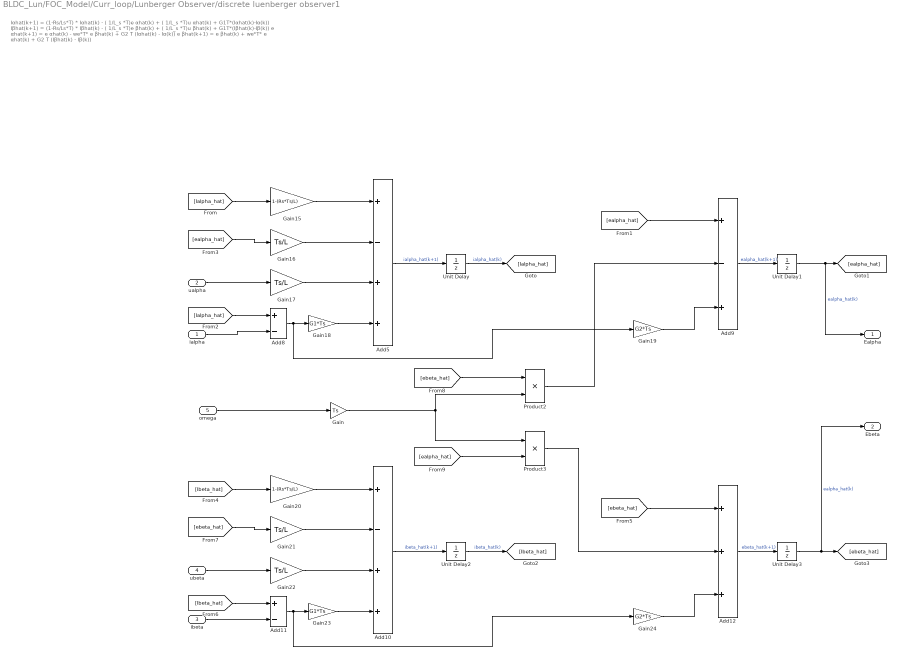
== system BLDC_Lun/FOC_Model/Curr_loop/Lunberger Observer/discrete luenberger observer1 ==
  note: Iαhat(k+1) = (1-Rs/Ls*T) * Iαhat(k) - ( 1/L_s *T)e αhat(k) + ( 1/L_s *T)u αhat(k) + G1T*(Iαhat(k)-Iα(k))
      | Iβhat(k+1) = (1-Rs/Ls*T) * Iβhat(k) - ( 1/L_s *T)e βhat(k) + ( 1/L_s *T)u βhat(k) + G1T*(Iβhat(k)-Iβ(k))
      | e αhat(k+1) = e αhat(k) - we*T* e βhat(k) + G2 T (Iαhat(k) - Iα(k))
      | e βhat(k+1) = e βhat(k) + we*T* e αhat(k) + G2 T (Iβhat(k) - Iβ(k))
  ialpha : Inport  OutDataTypeStr=single
  ualpha : Inport  Port=2  OutDataTypeStr=single
  ibeta : Inport  Port=3  OutDataTypeStr=single
  ubeta : Inport  Port=4  OutDataTypeStr=single
  omega : Inport  Port=5  OutDataTypeStr=single
  Add10 : Sum  Inputs=+-++
  Add11 : Sum  Inputs=+-
  Add12 : Sum  Inputs=+++
  Add5 : Sum  Inputs=+-++
  Add8 : Sum  Inputs=+-
  Add9 : Sum  Inputs=+-+
  Gain : Gain  Gain=Ts
  Gain15 : Gain  Gain=1-(Rs*Ts/L)
  Gain{16..17,21..22} (4 alike) : Gain  Gain=Ts/L
  Gain18 : Gain  Gain=G1*Ts
  Gain19 : Gain  Gain=G2*Ts
  Gain20 : Gain  Gain=1-(Rs*Ts/L)
  Gain23 : Gain  Gain=G1*Ts
  Gain24 : Gain  Gain=G2*Ts
  Product2 : Product
  Product3 : Product
  Unit Delay{,1..3} (4 alike) : UnitDelay  SampleTime=-1  HasFrameUpgradeWarning=on
  Ealpha : Outport
  Ebeta : Outport  Port=2
  wires:
  Add5/1 -> Unit Delay/1  "ialpha_hat(k+1)"
  Gain15/1 -> Add5/1
  Gain16/1 -> Add5/2
  Gain17/1 -> Add5/3
  Add8/1 -> Gain19/1, Gain18/1
  ialpha/1 -> Add8/2
  Gain18/1 -> Add5/4
  Unit Delay/1 -> [Ialpha_hat]  "ialpha_hat(k)"
  [Ialpha_hat] -> Gain15/1
  ualpha/1 -> Gain17/1
  [ealpha_hat] -> Gain16/1
  [Ialpha_hat] -> Add8/1
  Add9/1 -> Unit Delay1/1  "ealpha_hat(k+1)"
  Unit Delay1/1 -> Ealpha/1, [ealpha_hat]  "ealpha_hat(k)"
  [ealpha_hat] -> Add9/1
  Gain19/1 -> Add9/3
  ubeta/1 -> Gain22/1
  [ebeta_hat] -> Gain21/1
  [ebeta_hat] -> Add12/1
  Add11/1 -> Gain24/1, Gain23/1
  Unit Delay2/1 -> [Ibeta_hat]  "ibeta_hat(k)"
  Gain21/1 -> Add10/2
  Gain20/1 -> Add10/1
  Add10/1 -> Unit Delay2/1  "ibeta_hat(k+1)"
  Gain24/1 -> Add12/3
  Gain22/1 -> Add10/3
  Gain23/1 -> Add10/4
  [Ibeta_hat] -> Add11/1
  Add12/1 -> Unit Delay3/1  "ebeta_hat(k+1)"
  ibeta/1 -> Add11/2
  [Ibeta_hat] -> Gain20/1
  Unit Delay3/1 -> Ebeta/1, [ebeta_hat]  "ealpha_hat(k)"
  omega/1 -> Gain/1
  [ebeta_hat] -> Product2/1
  Gain/1 -> Product2/2, Product3/1
  Product2/1 -> Add9/2
  [ealpha_hat] -> Product3/2
  Product3/1 -> Add12/2

== system BLDC_Lun/FOC_Model/Curr_loop/SVPWM1/InvClark ==
  Valpha : Inport  OutDataTypeStr=single
  Vbeta : Inport  Port=2  OutDataTypeStr=single
  Gain : Gain  Gain=-1/2  OutDataTypeStr=single
  Gain1 : Gain  Gain=sqrt(3)/2  OutDataTypeStr=single
  Sum : Sum  Inputs=|++  OutDataTypeStr=single
  Sum1 : Sum  Inputs=-+|  OutDataTypeStr=single
  Va : Outport  OutDataTypeStr=single
  Vb : Outport  Port=2  OutDataTypeStr=single
  Vc : Outport  Port=3  OutDataTypeStr=single
  wires:
  Valpha/1 -> Gain/1, Va/1
  Vbeta/1 -> Gain1/1
  Gain/1 -> Sum1/2, Sum/1
  Sum/1 -> Vb/1
  Gain1/1 -> Sum/2, Sum1/1
  Sum1/1 -> Vc/1

== system BLDC_Lun/FOC_Model/Curr_loop/SVPWM1/ei_t ==
  Vabc : Inport  OutDataTypeStr=single
  Demux : Demux  Outputs=3
  Gain : Gain  Gain=-1/2  OutDataTypeStr=single
  Min : MinMax  Inputs=3  OutDataTypeStr=single
  Min1 : MinMax  Function=max  Inputs=3  OutDataTypeStr=single
  Sum : Sum  Inputs=|++  OutDataTypeStr=single
  ei_t : Outport  OutDataTypeStr=single
  wires:
  Min/1 -> Sum/1
  Sum/1 -> Gain/1
  Min1/1 -> Sum/2
  Gain/1 -> ei_t/1
  Vabc/1 -> Demux/1
  Demux/1 -> Min1/1, Min/1
  Demux/2 -> Min/2, Min1/2
  Demux/3 -> Min1/3, Min/3

== system BLDC_Lun/FOC_Model/Curr_loop/Lunberger Observer/PLL2/SpeedToTheta ==
  we : Inport
  Angle_Limit : Subsystem
  Sum1 : Sum  Inputs=|++
  Ts : Gain  Gain=1e-4
  Unit Delay : UnitDelay  SampleTime=-1  HasFrameUpgradeWarning=on
  Theta : Outport
  wires:
  we/1 -> Ts/1
  Ts/1 -> Sum1/1
  Sum1/1 -> Angle_Limit/1(Angle_input)
  Unit Delay/1 -> Theta/1, Sum1/2
  Angle_Limit/1(Angle_output) -> Unit Delay/1

== system BLDC_Lun/FOC_Model/Curr_loop/Lunberger Observer/PLL2/SpeedToTheta/Angle_Limit ==
  Angle_input : Inport
  If Action Subsystem1 : Subsystem  TreatAsAtomicUnit=on
  If Action Subsystem2 : Subsystem  TreatAsAtomicUnit=on
  If Action Subsystem3 : Subsystem  TreatAsAtomicUnit=on
  If1 : If  IfExpression=u1 > 6.283185307  ElseIfExpressions=u1<0
  Merge1 : Merge  Inputs=3
  Angle_output : Outport
  wires:
  If1/2 -> If Action Subsystem3/Action
  If1/1 -> If Action Subsystem2/Action
  If1/3 -> If Action Subsystem1/Action
  Merge1/1 -> Angle_output/1
  If Action Subsystem1/1(Out1) -> Merge1/3
  If Action Subsystem2/1(Out1) -> Merge1/1
  Angle_input/1 -> If Action Subsystem3/1(In1), If Action Subsystem1/1(In1), If Action Subsystem2/1(In1), If1/1
  If Action Subsystem3/1(Out1) -> Merge1/2

== system BLDC_Lun/FOC_Model/Curr_loop/Lunberger Observer/PLL2/SpeedToTheta/Angle_Limit/If Action Subsystem1 ==
  In1 : Inport
  Action Port : ActionPort  ActionPortLabel=else
  Out1 : Outport
  wires:
  In1/1 -> Out1/1

== system BLDC_Lun/FOC_Model/Curr_loop/Lunberger Observer/PLL2/SpeedToTheta/Angle_Limit/If Action Subsystem2 ==
  In1 : Inport
  Action Port : ActionPort  ActionPortLabel=if(u1 > 6.283185307)
  2pi : Constant  Value=2*pi  OutDataTypeStr=single
  Subtract1 : Sum  Inputs=+-  OutDataTypeStr=single
  Out1 : Outport
  wires:
  In1/1 -> Subtract1/1
  Subtract1/1 -> Out1/1
  2pi/1 -> Subtract1/2

== system BLDC_Lun/FOC_Model/Curr_loop/Lunberger Observer/PLL2/SpeedToTheta/Angle_Limit/If Action Subsystem3 ==
  In1 : Inport
  Action Port : ActionPort  ActionPortLabel=elseif(u1<0)
  Angle_offset : Constant  Value=2*pi  OutDataTypeStr=single
  Subtract1 : Sum
  Out1 : Outport
  wires:
  In1/1 -> Subtract1/1
  Subtract1/1 -> Out1/1
  Angle_offset/1 -> Subtract1/2

== matlab function BLDC_Lun/FOC_Model/Curr_loop/svpwm2 ==
  data: Valpha input; Tcmp1 output; Vbeta input; Udc input; Tpwm input; Tcmp2 output; Tcmp3 output; sector output
function [Tcmp1,Tcmp2,Tcmp3,sector] = fcn(Valpha,Vbeta,Udc,Tpwm)
%#codegen

sector = single(0);
Tcmp1 = single(0);
Tcmp2 = single(0);
Tcmp3 = single(0);

%========Parameters statement================

    Vref1 = Vbeta;							                   
    Vref2 = (sqrt(3)*Valpha - Vbeta)/2; 				    
    Vref3 = (-sqrt(3)*Valpha - Vbeta)/2;					
   
 %========Sector calculation=================

  if (Vref1>0)
	   sector = single(1);
  end
  if (Vref2>0)
	   sector = sector+single(2);
  end
  if (Vref3>0)
       sector = sector+single(4);
  end

%======== X Y Z calculation===================

X = sqrt(3)*Vbeta*Tpwm/Udc;
Y = Tpwm/Udc*(3/2*Valpha+sqrt(3)/2*Vbeta);
Z = Tpwm/Udc*(-3/2*Valpha+sqrt(3)/2*Vbeta);	         

%==========Duty ratio calculation================
switch (sector)   
    case 1
        T1 = Z; T2 = Y; 
	case 2
        T1 = Y; T2 = -X; 
	case 3
        T1 = -Z; T2 = X; 
	case 4
        T1 = -X; T2 = Z;
	case 5
        T1 = X; T2 = -Y;
    otherwise
        T1 = -Y; T2 = -Z;
end

if T1+T2 > Tpwm
    T1 = T1/(T1+T2);
    T2 = T2/(T1+T2);
else
    T1 = T1;
    T2 = T2;
end
ta = (Tpwm-(T1+T2))/4.0;
tb = ta+T1/2;
tc = tb+T2/2;

%==========Duty ratio calculation================
switch (sector)
    case 1 
        Tcmp1=tb;
        Tcmp2=ta;
        Tcmp3=tc; 
        
    case 2 
        Tcmp1=ta;
        Tcmp2=tc;
        Tcmp3=tb; 
       
    case 3 
        Tcmp1=ta;
        Tcmp2=tb;
        Tcmp3=tc; 
        
    case 4 
        Tcmp1=tc;
        Tcmp2=tb;
        Tcmp3=ta;
        
    case 5 
        Tcmp1=tc;
        Tcmp2=ta;
        Tcmp3=tb;
        
   case 6
       Tcmp1=tb;
       Tcmp2=tc;
       Tcmp3=ta;
end
end

== stateflow chart BLDC_Lun/FOC_Model/Curr_loop/Chart1 ==
  state OpenStage
    en:
    ZReset = 0;
    cnt = 0;
    du:
    if cnt == 1
    ZReset = 1;
    end
    cnt = 1;
    Motor_state = 3;
    RestsSingal = 0;
  state IDLE
    en:
    du:
    Motor_state = 1;
    RestsSingal = 0;
  state AlignStage
    en:
    du:
    Motor_state = 2;
    RestsSingal = 0;
  state ThetaAlign
    en:
    du:
    Motor_state = 4;
    RestsSingal = 0;
  state RunStage
    en:
    du:
    Motor_state = 5;
    RestsSingal = 1;
  (default) -> IDLE
  IDLE -> AlignStage : [Motor_OnOff ==1]
  AlignStage -> OpenStage [order 1] : [after(1000,tick)]
  OpenStage -> ThetaAlign [order 2] : [after(30000,tick) ]
  ThetaAlign -> RunStage : [after(5000,tick)]
  AlignStage -> IDLE [order 2] : [Motor_OnOff == 0]
  RunStage -> IDLE : [Motor_OnOff ==0]
  OpenStage -> IDLE [order 1] : [Motor_OnOff ==0]
  data: Motor_OnOff input; Motor_state output single; RestsSingal output; ZReset output single; cnt local single
